simulink model "PID_model_comparison"  (R2023a)
settings: Solver=FixedStepAuto  StartTime=0.0  StopTime=10  FixedStep=Ts  RelTol=1e-3  EnableMultiTasking=on
PreLoadFcn:
  | load('ModelParameters.mat')
StartFcn:
  | Ts=0.03
libraries: slpidlib x1
settings Model: ExtModeTrigDuration=5  Creator=AlexandrY  LastModifiedBy=DeveloperY
settings SolverCC: AlgebraicLoopSolver=TrustRegion  AutoInsertRateTranBlk=on
settings DataIOCC: ReturnWorkspaceOutputs=off
settings OptimizationCC: DefaultParameterBehavior=Inlined  UseDivisionForNetSlopeComputation=on  UseFloatMulNetSlope=on  InlineInvariantSignals=on  PassReuseOutputArgsAs=Individual arguments  ZeroExternalMemoryAtStartup=off  ZeroInternalMemoryAtStartup=off  NoFixptDivByZeroProtection=on  EfficientFloat2IntCast=on  LifeSpan=1  MaxStackSize=64  EfficientTunableParamExpr=on
settings DebuggingCC: ParameterTunabilityLossMsg=error  UnconnectedInputMsg=warning  UnconnectedOutputMsg=warning  UnconnectedLineMsg=warning  BusObjectLabelMismatch=error  ArithmeticOperatorsInVariantConditions=warning
settings HardwareCC: ProdBitPerPointer=32  ProdBitPerSizeT=32  ProdBitPerPtrDiffT=32  ProdLargestAtomicInteger=Long  ProdLargestAtomicFloat=Double  ProdWordSize=32  ProdHWDeviceType=ARM Compatible->ARM Cortex
settings ModelReferenceCC: EnableRefExpFcnMdlSchedulingChecks=on
settings SFSimCC: SimUseLocalCustomCode=off  MATLABDynamicMemAlloc=off  CustomCodeUndefinedFunction=UseInterfaceOnly
settings RTWCC: Description=Embedded Coder  SystemTargetFile=ert.tlc  HardwareBoard=NXP FRDM-K64F  TLCOptions="-aInlineSetEventsForThisBaseRateFcn=TLC_FALSE -aSuppressMultiTaskScheduler=TLC_FALSE  -aRateBasedStepFcn=0"  PackageGeneratedCodeAndArtifacts=on  PackageName=GeneratedCode  TemplateMakefile=ert_default_tmf  GenerateReport=on  RTWUseLocalCustomCode=off  Toolchain=GNU Tools for ARM Embedded Processors  BuildConfiguration=Debug  IncludeHyperlinkInReport=on  LaunchReport=on  GenerateTraceInfo=on  GenerateTraceReport=on  GenerateTraceReportSl=on  GenerateTraceReportSf=on  GenerateTraceReportEml=on  GenerateCodeMetricsReport=on
settings CodeAppCC: ForceParamTrailComments=on  CommentStyle=Single-line  IgnoreCustomStorageClasses=off  OperatorAnnotations=on  SimulinkDataObjDesc=on  SFDataObjDesc=on  MATLABFcnDesc=on  CustomSymbolStrGlobalVar=rt$N$M  CustomSymbolStrType=$N$M  CustomSymbolStrFcn=$N$M$F  CustomSymbolStrMacro=$N$M  InsertBlockDesc=on  StateflowObjectComments=on  MATLABSourceComments=on  EnableCustomComments=on  ReqsInCode=on
settings ERTTargetCC: CodeReplacementLibrary=ARM Cortex-M (Optimized)  MultiwordLength=2048  IncludeMdlTerminateFcn=off  CombineSignalStateStructs=on  CodeInterfacePackaging=Reusable function  SupportComplex=off  SupportNonInlinedSFcns=on  ParenthesesLevel=Maximum  InlinedParameterPlacement=NonHierarchical  RootIOFormat=Structure reference  ERTFilePackagingFormat=CompactWithDataFile  ConvertIfToSwitch=off  IndentStyle=Allman

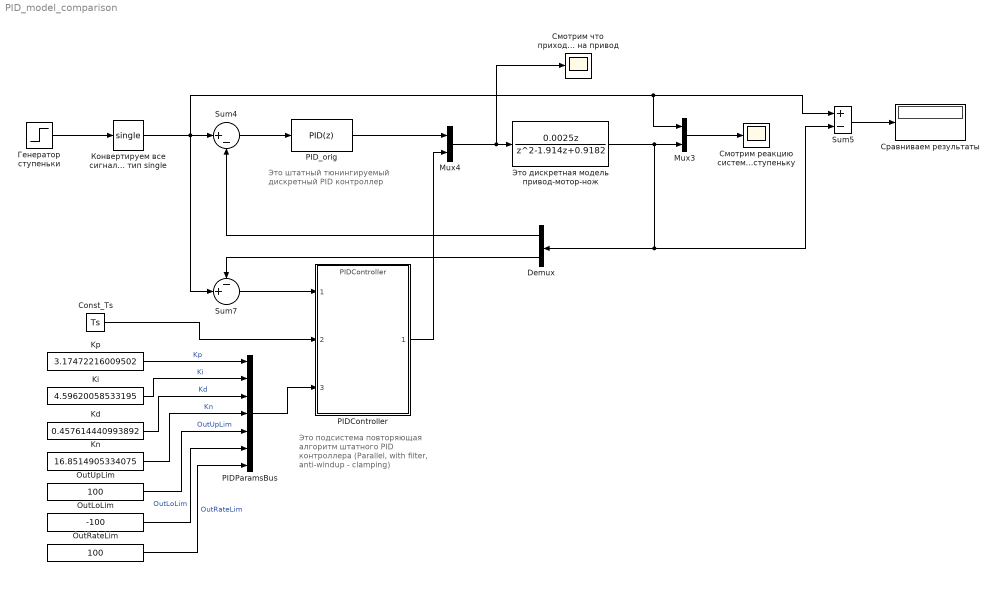
== system PID_model_comparison ==
  note: Это подсистема повторяющая
      | алгоритм штатного
      | PID контроллера (Parallel, with filter, anti-windup - clamping)
  note: Это штатный тюнингируемый
      | дискретный PID контроллер
  Const_Ts : Constant  DisableCoverage=on  Value=Ts  OutDataTypeStr=single  SampleTime=-1  PreserveConstantTs=on
  Demux : Demux  Outputs=2
  Kd : Constant  DisableCoverage=on  Value=0.457614440993892  OutDataTypeStr=Inherit: Inherit via back propagation  SampleTime=Ts  PreserveConstantTs=on
  Ki : Constant  DisableCoverage=on  Value=4.59620058533195  OutDataTypeStr=Inherit: Inherit via back propagation  SampleTime=Ts  PreserveConstantTs=on
  Kn : Constant  DisableCoverage=on  Value=16.8514905334075  OutDataTypeStr=Inherit: Inherit via back propagation  SampleTime=Ts  PreserveConstantTs=on
  Kp : Constant  DisableCoverage=on  Value=3.17472216009502  OutDataTypeStr=Inherit: Inherit via back propagation  SampleTime=Ts  PreserveConstantTs=on
  Mux3 : Mux  Inputs=2
  Mux4 : Mux  Inputs=2
  OutLoLim : Constant  DisableCoverage=on  Value=-100  OutDataTypeStr=Inherit: Inherit via back propagation  SampleTime=Ts  PreserveConstantTs=on
  OutRateLim : Constant  DisableCoverage=on  Value=100  OutDataTypeStr=Inherit: Inherit via back propagation  SampleTime=Ts  PreserveConstantTs=on
  OutUpLim : Constant  DisableCoverage=on  Value=100  OutDataTypeStr=Inherit: Inherit via back propagation  SampleTime=Ts  PreserveConstantTs=on
  PIDController : ModelReference  ModelNameDialog=PIDController  SimulationMode=Normal  ModelReferenceVersion=12.0
  PIDParamsBus : BusCreator  Inputs='Kp','Ki','Kd','Kn','OutUpLim','OutLoLim','OutRateLim'  OutDataTypeStr=Bus: PIDParams
  PID_orig : slpidlib/PID Controller  Controller=PID  Form=Parallel  TimeDomain=Discrete-time  UseExternalTs=off  SampleTime=-1  IntegratorMethod=Forward Euler  FilterMethod=Forward Euler  ControllerParametersSource=internal  P=3.17472216009502  I=4.59620058533195  UseKiTs=off  D=0.457614440993892  N=16.8514905334075  UseFilter=on  TunerSelectOption=Transfer Function Based (PID Tuner App)  InitialConditionSource=internal  InitialConditionForIntegrator=0  InitialConditionForFilter=0  DifferentiatorICPrevScaledInput=0  ExternalReset=none  TrackingMode=off  Kt=1  LimitOutput=on  SatLimitsSource=internal  UpperSaturationLimit=100  LowerSaturationLimit=-100  LinearizeAsGain=off  AntiWindupMode=clamping  Kb=4  LimitIntegrator=off  UpperIntegratorSaturationLimit=inf  LowerIntegratorSaturationLimit=-inf  PGainOutDataTypeStr=single  PProdOutDataTypeStr=single  POutMin=[]  POutMax=[]  IGainOutDataTypeStr=single  IProdOutDataTypeStr=single  IOutMin=[]  IOutMax=[]  DGainOutDataTypeStr=single  DProdOutDataTypeStr=single  DOutMin=[]  DOutMax=[]  NGainOutDataTypeStr=single  NProdOutDataTypeStr=single  NOutMin=[]  NOutMax=[]  SumOutDataTypeStr=single  SumOutMin=[]  SumOutMax=[]  SaturationOutMin=[]  SaturationOutMax=[]  PParamDataTypeStr=single  PParamMin=[]  PParamMax=[]  IParamDataTypeStr=single  IParamMin=[]  IParamMax=[]  DParamDataTypeStr=single  DParamMin=[]  DParamMax=[]  NParamDataTypeStr=single  NParamMin=[]  NParamMax=[]  KbParamMin=[]  KbParamMax=[]  KtParamMin=[]  KtParamMax=[]  KbOutMin=[]  KbOutMax=[]  KtOutMin=[]  KtOutMax=[]  IntegratorOutDataTypeStr=single  IntegratorOutMin=[]  IntegratorOutMax=[]  FilterOutDataTypeStr=single  FilterOutMin=[]  FilterOutMax=[]  SumI1OutMin=[]  SumI1OutMax=[]  SumI2OutMin=[]  SumI2OutMax=[]  SumI3OutMin=[]  SumI3OutMax=[]  SumI4OutMin=[]  SumI4OutMax=[]  SumDOutDataTypeStr=single  SumDOutMin=[]  SumDOutMax=[]  SumAccumDataTypeStr=single  SumDAccumDataTypeStr=single  DifferentiatorOutMin=[]  DifferentiatorOutMax=[]  FilterDiffOutCoefMin=[]  FilterDiffOutCoefMax=[]  ReciprocalOutMin=[]  ReciprocalOutMax=[]  SumDenOutMin=[]  SumDenOutMax=[]  SumNumOutMin=[]  SumNumOutMax=[]  DivideOutMin=[]  DivideOutMax=[]  UdiffTsProdOutMin=[]  UdiffTsProdOutMax=[]  NTsProdOutMin=[]  NTsProdOutMax=[]  UintegralTsProdOutMin=[]  UintegralTsProdOutMax=[]  UngainTsProdOutMin=[]  UngainTsProdOutMax=[]  ClampingZeroOutDataTypeStr=Inherit: Inherit via back propagation  ClampingZeroOutMin=[]  ClampingZeroOutMax=[]  FilterDenConstantOutDataTypeStr=Inherit: Inherit via back propagation  FilterDenConstantOutMin=[]  FilterDenConstantOutMax=[]  PCopyOutDataTypeStr=Inherit: Inherit via back propagation  PCopyOutMin=[]  PCopyOutMax=[]  NCopyOutDataTypeStr=Inherit: Inherit via back propagation  NCopyOutMin=[]  NCopyOutMax=[]  IntegratorContinuousStateAttributes=''  IntegratorStateMustResolveToSignalObject=off  IntegratorRTWStateStorageClass=Auto  FilterContinuousStateAttributes=''  FilterStateMustResolveToSignalObject=off  FilterRTWStateStorageClass=Auto  ParallelPVariant=InternalParameters  IdealPVariant=Disabled  IVariant=InternalParameters  DVariant=InternalParameters  IntegratorVariant=Discrete  SatVariant=Enabled  AWVariant=DiscClampingParallel  PCopyVariant=Disabled  TRVariant=Disabled  FdbkBlocksVariant=Forward  IdealPFdbkVariant=Disabled  SatFdbkVariant=Disabled  DerivativeFilterVariant=ForwardEulerFilter  NVariant=InternalParameters  NCopyVariant=Disabled  FilterICVariant=InternalICsFilter  IntegratorICVariant=InternalICs  ExternalResetVariant=Disabled  TRSumVariant=Passthrough  SumFdbkVariant=Disabled  SumVariant=Sum_PID  TsampFilterVariant=InternalTs  TsampNgainVariant=Passthrough  TsampIntegralVariant=Disabled_SignalSpec  ExternalSaturationOutDataTypeStr=Inherit: Same as second input
  Sum4 : Sum  Inputs=|+-
  Sum5 : Sum  Inputs=+-
  Sum7 : Sum  Inputs=-+|
  Генератор ступеньки : Step  After=15  SampleTime=Ts
  "Конвертируем все сигналы модели в тип single " : DataTypeConversion  OutDataTypeStr=single  SaturateOnIntegerOverflow=off  RndMeth=Floor
  Смотрим реакцию системы на ступеньку : Scope
  Смотрим что приходит на привод : Scope
  "Сравниваем результаты " : Display
  Это дискретная модель привод-мотор-нож : DiscreteTransferFcn  Numerator=[0.0025 0]  Denominator=[1 -1.914 0.9182]
  wires:
  Генератор ступеньки/1 -> "Конвертируем все сигналы модели в тип single "/1
  Sum4/1 -> PID_orig/1
  PID_orig/1 -> Mux4/1
  "Конвертируем все сигналы модели в тип single "/1 -> Sum5/1, Mux3/1, Sum7/2, Sum4/1
  Это дискретная модель привод-мотор-нож/1 -> Mux3/2, Demux/1, Sum5/2
  Mux3/1 -> Смотрим реакцию системы на ступеньку/1
  Sum5/1 -> "Сравниваем результаты "/1
  Mux4/1 -> Это дискретная модель привод-мотор-нож/1, Смотрим что приходит на привод/1
  Demux/1 -> Sum4/2
  Sum7/1 -> PIDController/1
  PIDController/1 -> Mux4/2
  Demux/2 -> Sum7/1
  Kp/1 -> PIDParamsBus/1  "Kp"
  Ki/1 -> PIDParamsBus/2  "Ki"
  Kd/1 -> PIDParamsBus/3  "Kd"
  Kn/1 -> PIDParamsBus/4  "Kn"
  OutUpLim/1 -> PIDParamsBus/5  "OutUpLim"
  OutLoLim/1 -> PIDParamsBus/6  "OutLoLim"
  OutRateLim/1 -> PIDParamsBus/7  "OutRateLim"
  PIDParamsBus/1 -> PIDController/3
  Const_Ts/1 -> PIDController/2
